simulink model "WT_pitch_actuator_no_sat"  (R2024a)
settings: Solver=FixedStepAuto  StartTime=0.0  StopTime=10.0  FixedStep=0.001  RelTol=1e-3
settings Model: Creator=ml4  LastModifiedBy=ml4

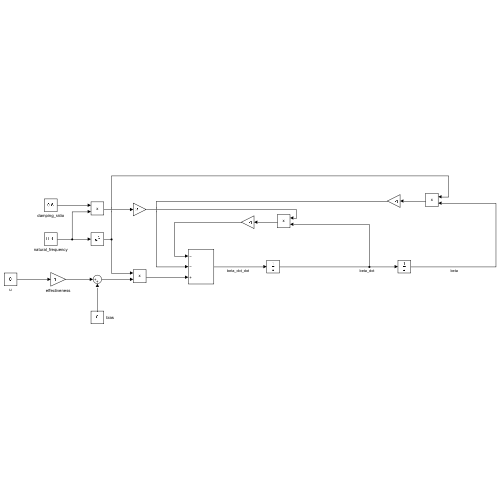
[thumbnail: Simulink's stored preview of the top-level diagram]
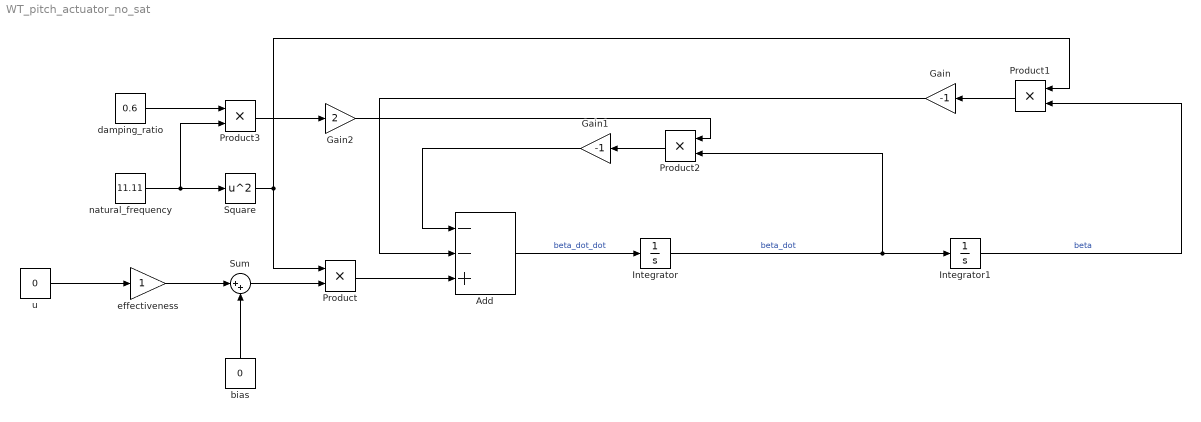
== system WT_pitch_actuator_no_sat ==
  Add : Sum  Inputs=--+
  Gain : Gain  Gain=-1
  Gain1 : Gain  Gain=-1
  Gain2 : Gain  Gain=2
  Integrator : Integrator
  Integrator1 : Integrator
  Product{,1..3} (4 alike) : Product
  Square : Math  Operator=square
  Sum : Sum  Inputs=|++
  bias : Constant  Value=0
  damping_ratio : Constant  Value=0.6
  effectiveness : Gain
  natural_frequency : Constant  Value=11.11
  u : Constant  Value=0
  wires:
  Gain/1 -> Add/2
  Gain2/1 -> Product2/1
  damping_ratio/1 -> Product3/1
  Square/1 -> Product1/1, Product/1
  Sum/1 -> Product/2
  natural_frequency/1 -> Product3/2, Square/1
  bias/1 -> Sum/2
  effectiveness/1 -> Sum/1
  Product2/1 -> Gain1/1
  Product1/1 -> Gain/1
  Integrator/1 -> Product2/2, Integrator1/1  "beta_dot"
  Add/1 -> Integrator/1  "beta_dot_dot"
  Gain1/1 -> Add/1
  Product/1 -> Add/3
  u/1 -> effectiveness/1
  Product3/1 -> Gain2/1
  Integrator1/1 -> Product1/2  "beta"
